simulink model "SildeModel_control"  (R2022b)
settings: Solver=ode4  StartTime=0.0  StopTime=t_total  FixedStep=sim_dt  RelTol=1e-3  EnableMultiTasking=on
InitFcn:
  | InitialCondition
values from neighbouring files (symbols this model uses):
  eps1 = 1e-4    (= 0.0001)    [InitialCondition.m]    (also in precise_plot.m = eps1_list(k))
  I_B = diag([200, 250, 300])    [InitialCondition.m]
  I_B_REAL = I_B*1.05    [InitialCondition.m]
  lambda_max_J = max(eig(I_B))    [InitialCondition.m]
  mrp0 = [0.2, 0.3, -0.3]    [InitialCondition.m]
  MRP_last = MRP_SEQ(end,:)    [InitialCondition.m]
  MRP_REAL0 = MRP_REAL0'    [InitialCondition.m]
  sim_dt = 0.01    [InitialCondition.m]
  Tau_SEQ = [Tau_SEQ;   Tau_EXT]    [InitialCondition.m]
  w0 = w0(:)    [Gauss_opt_mrp.m]    (also in InitialCondition.m = [0; 0; 0])
settings Model: Creator=Administrator  LastModifiedBy=33592
settings DataIOCC: ExternalInput=[t, y]  LimitDataPoints=on  MaxDataPoints=15000  ReturnWorkspaceOutputs=off
settings OptimizationCC: LifeSpan=inf
settings DebuggingCC: MultiTaskCondExecSysMsg=warning  MultiTaskRateTransMsg=warning  UnconnectedInputMsg=warning  UnconnectedOutputMsg=warning  UnconnectedLineMsg=warning  AllowSymbolicDim=off  SFUnexpectedBacktrackingDiag=warning  SFNoUnconditionalDefaultTransitionDiag=warning  SFExecutionAtInitializationDiag=none  SFMachineParentedDataDiag=warning  ArithmeticOperatorsInVariantConditions=warning
settings ModelReferenceCC: EnableRefExpFcnMdlSchedulingChecks=on  PropagateSignalLabelsOutOfModel=off
settings SFSimCC: SimUseLocalCustomCode=off  CustomCodeUndefinedFunction=UseInterfaceOnly
settings RTWCC: RTWUseLocalCustomCode=off
settings CodeAppCC: StateflowObjectComments=on
settings GRTTargetCC: TargetLangStandard=C89/C90 (ANSI)
settings ConfigComp: CovMetricSettings=dw  CovSaveCumulativeToWorkspaceVar=on  CovSaveSingleToWorkspaceVar=on  CovExternalEMLEnable=off

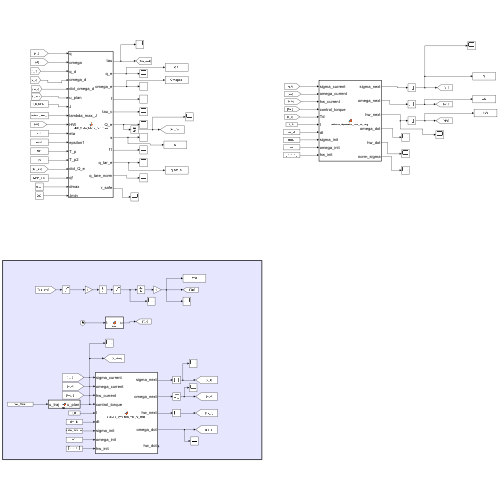
[thumbnail: Simulink's stored preview of the top-level diagram]
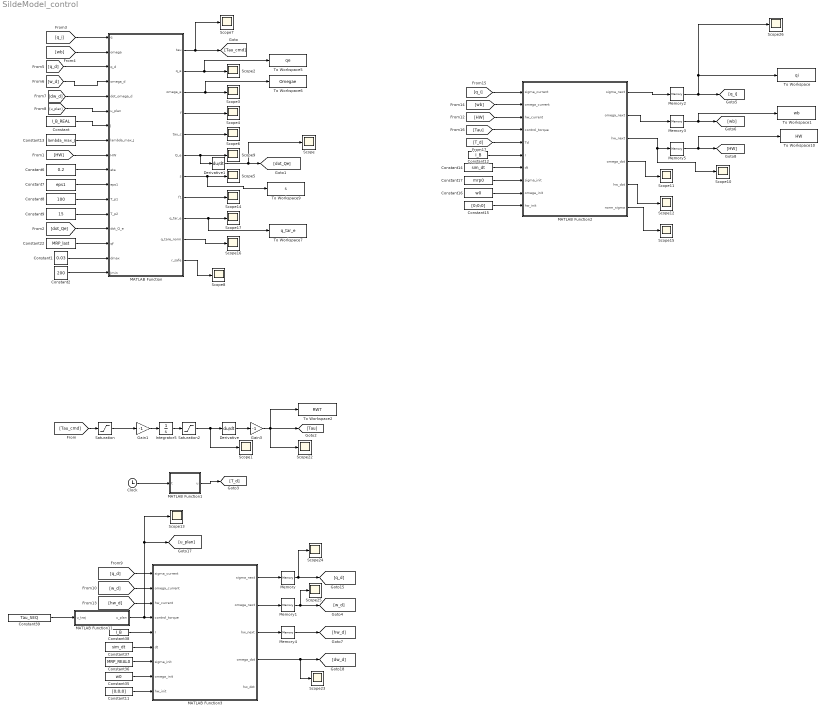
== system SildeModel_control ==
  Clock : Clock
  Constant : Constant  Value=I_B_REAL
  Constant1 : Constant  Value=0.03
  Constant11 : Constant  Value=[0;0;0]
  Constant12 : Constant  Value=I_B
  Constant13 : Constant  Value=lambda_max_J
  Constant14 : Constant  Value=sim_dt
  Constant15 : Constant  Value=[0;0;0]
  Constant16 : Constant  Value=w0
  Constant17 : Constant  Value=mrp0
  Constant2 : Constant  Value=200
  Constant22 : Constant  Value=MRP_last
  Constant35 : Constant  Value=w0
  Constant36 : Constant  Value=MRP_REAL0
  Constant37 : Constant  Value=sim_dt
  Constant38 : Constant  Value=I_B
  Constant39 : Constant  Value=Tau_SEQ
  Constant6 : Constant  Value=0.2
  Constant7 : Constant  Value=eps1
  Constant8 : Constant  Value=100
  Constant9 : Constant  Value=15
  Derivative : Derivative
  Derivative1 : Derivative
  Gain1 : Gain  Gain=-1
  Gain3 : Gain  Gain=-1
  Integrator5 : Integrator
  MATLAB Function : MATLAB Function  TreatAsAtomicUnit=on
  MATLAB Function1 : MATLAB Function  TreatAsAtomicUnit=on
  MATLAB Function11 : MATLAB Function  TreatAsAtomicUnit=on
  MATLAB Function2 : MATLAB Function  TreatAsAtomicUnit=on
  MATLAB Function3 : MATLAB Function  TreatAsAtomicUnit=on
  Memory{,1..5} (6 alike) : Memory
  Saturation : Saturate  UpperLimit=0.2  LowerLimit=-0.2
  Saturation2 : Saturate  UpperLimit=4  LowerLimit=-4
  Scope{,1..17,22..26} (23 alike) : Scope
  To Workspace : ToWorkspace  VariableName=qi  SampleTime=-1
  To Workspace1 : ToWorkspace  VariableName=wb  SampleTime=-1
  To Workspace10 : ToWorkspace  VariableName=HW  SampleTime=-1
  To Workspace2 : ToWorkspace  VariableName=RWT  SampleTime=-1
  To Workspace5 : ToWorkspace  VariableName=qe  SampleTime=-1
  To Workspace6 : ToWorkspace  VariableName=Omegae  SampleTime=-1
  To Workspace7 : ToWorkspace  VariableName=q_tar_e  SampleTime=-1
  To Workspace9 : ToWorkspace  VariableName=s  SampleTime=-1
  wires:
  MATLAB Function/1(tau) -> Scope7/1, [Tau_cmd]
  [q_i] -> MATLAB Function/1(q)
  [wb] -> MATLAB Function/2(omega)
  Constant/1 -> MATLAB Function/7(J)
  MATLAB Function/2(q_e) -> To Workspace5/1, Scope2/1
  Constant6/1 -> MATLAB Function/10(eta)
  Constant7/1 -> MATLAB Function/11(eps1)
  Constant8/1 -> MATLAB Function/12(T_p1)
  Constant9/1 -> MATLAB Function/13(T_p2)
  MATLAB Function/3(omega_e) -> To Workspace6/1, Scope3/1
  MATLAB Function/4(f) -> Scope4/1
  Constant13/1 -> MATLAB Function/8(lambda_max_J)
  MATLAB Function/7(s) -> To Workspace9/1, Scope5/1
  MATLAB Function/5(tau_c) -> Scope6/1
  MATLAB Function/6(Q_e) -> Derivative1/1, Scope9/1
  Clock/1 -> MATLAB Function1/1(t)
  MATLAB Function1/1(u) -> [T_d]
  MATLAB Function/8(f1) -> Scope14/1
  Constant22/1 -> MATLAB Function/15(qf)
  MATLAB Function/9(q_tar_e) -> To Workspace7/1, Scope17/1
  Gain1/1 -> Integrator5/1
  Constant35/1 -> MATLAB Function3/8(omega_init)
  Constant36/1 -> MATLAB Function3/7(sigma_init)
  Constant37/1 -> MATLAB Function3/6(dt)
  Constant38/1 -> MATLAB Function3/5(I)
  Constant39/1 -> MATLAB Function11/1(u_traj)
  MATLAB Function11/1(u_plan) -> Scope13/1, [u_plan], MATLAB Function3/4(control_torque)
  MATLAB Function3/1(sigma_next) -> Memory/1
  Memory/1 -> [q_d], Scope24/1
  MATLAB Function3/2(omega_next) -> Memory1/1
  Memory1/1 -> [w_d], Scope25/1
  MATLAB Function3/4(omega_dot) -> Scope23/1, [dw_d]
  MATLAB Function3/3(hw_next) -> Memory4/1
  Memory4/1 -> [hw_d]
  [q_d] -> MATLAB Function3/1(sigma_current)
  [w_d] -> MATLAB Function3/2(omega_current)
  [hw_d] -> MATLAB Function3/3(hw_current)
  Constant11/1 -> MATLAB Function3/9(hw_init)
  MATLAB Function2/1(sigma_next) -> Memory2/1
  Memory3/1 -> To Workspace1/1, [wb]
  Memory2/1 -> [q_i], To Workspace/1, Scope26/1
  MATLAB Function2/2(omega_next) -> Memory3/1
  MATLAB Function2/3(hw_next) -> Scope10/1, Memory5/1
  MATLAB Function2/4(omega_dot) -> Scope11/1
  MATLAB Function2/5(hw_dot) -> Scope12/1
  Memory5/1 -> To Workspace10/1, [HW]
  [HW] -> MATLAB Function2/3(hw_current)
  [wb] -> MATLAB Function2/2(omega_current)
  [q_i] -> MATLAB Function2/1(sigma_current)
  [Tau] -> MATLAB Function2/4(control_torque)
  [T_d] -> MATLAB Function2/5(Td)
  Constant12/1 -> MATLAB Function2/6(I)
  Constant14/1 -> MATLAB Function2/7(dt)
  Constant17/1 -> MATLAB Function2/8(sigma_init)
  Constant16/1 -> MATLAB Function2/9(omega_init)
  Constant15/1 -> MATLAB Function2/10(hw_init)
  [HW] -> MATLAB Function/9(HW)
  Derivative/1 -> Gain3/1
  Gain3/1 -> [Tau], To Workspace2/1, Scope22/1
  [u_plan] -> MATLAB Function/6(u_plan)
  [w_d] -> MATLAB Function/4(omega_d)
  [dw_d] -> MATLAB Function/5(dot_omega_d)
  [Tau_cmd] -> Saturation/1
  Saturation/1 -> Gain1/1
  Integrator5/1 -> Saturation2/1
  Derivative1/1 -> Scope/1, [dot_Qe]
  [dot_Qe] -> MATLAB Function/14(dot_Q_e)
  MATLAB Function/11(r_safe) -> Scope8/1
  Saturation2/1 -> Scope1/1, Derivative/1
  [q_d] -> MATLAB Function/3(q_d)
  Constant1/1 -> MATLAB Function/16(dmax)
  Constant2/1 -> MATLAB Function/17(Jmin)
  MATLAB Function2/6(norm_sigma) -> Scope15/1
  MATLAB Function/10(q_tare_norm) -> Scope16/1

== matlab function SildeModel_control/MATLAB Function3 ==
  data: sigma_current input; sigma_next output; omega_current input; hw_current input; control_torque input; I input; dt input; omega_next output; hw_next output; omega_dot output; sigma_init input; omega_init input; hw_init input; hw_dot output
function [sigma_next, omega_next, hw_next, omega_dot, hw_dot] = attitude_dynamics_mrp_rw_step(...
    sigma_current, omega_current, hw_current, control_torque, I, dt, sigma_init, omega_init, hw_init)
% 单步MRP姿态动力学计算（含反作用飞轮）- 用于Simulink
% 输入:
%   sigma_current - 当前MRP [σ1, σ2, σ3] (3×1)
%   omega_current - 当前角速度 [ω1, ω2, ω3] (3×1)
%   hw_current - 当前飞轮角动量 [hw1, hw2, hw3] (3×1)
%   control_torque - 控制力矩 [u1, u2, u3] (3×1) = -ḣw
%   I - 转动惯量矩阵 (3×3)
%   dt - 时间步长
%   reset - 重置信号，当为true时使用初始值
%   sigma_init - 初始MRP [σ1, σ2, σ3] (3×1)
%   omega_init - 初始角速度 [ω1, ω2, ω3] (3×1)
%   hw_init - 初始飞轮角动量 [hw1, hw2, hw3] (3×1)
% 输出:
%   sigma_next - 下一步MRP (3×1)
%   omega_next - 下一步角速度 (3×1)
%   hw_next - 下一步飞轮角动量 (3×1)
%   omega_dot - 当前角加速度 (3×1)
%   hw_dot - 当前飞轮角动量变化率 (3×1)
%   q_out - 对应的四元数 [q1, q2, q3, q4] (4×1)，用于参考
%   is_initialized - 初始化标志

    persistent initialized;
    
    % 第一次调用时初始化persistent变量
    if isempty(initialized)
        initialized = false;
    end
    
    % MRP动力学微分方程
    function dsigma = mrp_derivative(sigma, omega)
        % MRP运动学方程: σ̇ = G(σ)ω
        sigma_sq = sigma' * sigma;
        sigma_tilde = [0, -sigma(3), sigma(2); 
                      sigma(3), 0, -sigma(1);
                      -sigma(2), sigma(1), 0];
        
        G = 0.25 * ((1 - sigma_sq) * eye(3) + 2 * sigma_tilde + 2 * (sigma * sigma'));
        dsigma = G * omega;
    end

    % 角速度动力学微分方程（含飞轮）
    function dw = angular_velocity_derivative_rw(w, hw, u, I_matrix)
        % 欧拉动力学方程（含飞轮）: Iω̇ = u - ω × (Iω + hw)
        % 其中 u = -ḣw 是飞轮控制力矩
        dw = I_matrix \ (u - cross(w, I_matrix * w + hw));
    end

    % 飞轮角动量动力学微分方程
    function dhw = wheel_momentum_derivative(u)
        % 飞轮动力学: ḣw = -u
        % 其中 u = -ḣw 是飞轮控制力矩
        dhw = -u;
    end

    % 检查是否需要切换到影子MRP
    function sigma_checked = check_shadow_mrp(sigma)
        sigma_sq = sigma' * sigma;
        if sigma_sq > 1
            % 切换到影子MRP
            sigma_checked = -sigma / sigma_sq;
        else
            sigma_checked = sigma;
        end
    end

    % 处理初始化和重置
    if ~initialized
        % 使用初始值
        current_sigma = sigma_init(:);
        current_w = omega_init(:);
        current_hw = hw_init(:);
        initialized = true;
        is_initialized = true;
    else
        % 使用当前状态
        current_sigma = sigma_current(:);
        current_w = omega_current(:);
        current_hw = hw_current(:);
        is_initialized = false;
    end
    
    current_u = control_torque(:);
    
    % 计算角加速度和飞轮角动量变化率（用于输出）
    omega_dot = angular_velocity_derivative_rw(current_w, current_hw, current_u, I);
    hw_dot = wheel_momentum_derivative(current_u);
    
    % 使用四阶龙格-库塔法进行一步积分
    % k1
    k1_sigma = mrp_derivative(current_sigma, current_w);
    k1_w = angular_velocity_derivative_rw(current_w, current_hw, current_u, I);
    k1_hw = wheel_momentum_derivative(current_u);
    
    % k2
    k2_sigma = mrp_derivative(current_sigma + 0.5 * dt * k1_sigma, current_w + 0.5 * dt * k1_w);
    k2_w = angular_velocity_derivative_rw(current_w + 0.5 * dt * k1_w, current_hw + 0.5 * dt * k1_hw, current_u, I);
    k2_hw = wheel_momentum_derivative(current_u);
    
    % k3
    k3_sigma = mrp_derivative(current_sigma + 0.5 * dt * k2_sigma, current_w + 0.5 * dt * k2_w);
    k3_w = angular_velocity_derivative_rw(current_w + 0.5 * dt * k2_w, current_hw + 0.5 * dt * k2_hw, current_u, I);
    k3_hw = wheel_momentum_derivative(current_u);
    
    % k4
    k4_sigma = mrp_derivative(current_sigma + dt * k3_sigma, current_w + dt * k3_w);
    k4_w = angular_velocity_derivative_rw(current_w + dt * k3_w, current_hw + dt * k3_hw, current_u, I);
    k4_hw = wheel_momentum_derivative(current_u);
    
    % 更新MRP、角速度和飞轮角动量
    next_sigma = current_sigma + (dt / 6) * (k1_sigma + 2*k2_sigma + 2*k3_sigma + k4_sigma);
    next_w = current_w + (dt / 6) * (k1_w + 2*k2_w + 2*k3_w + k4_w);
    next_hw = current_hw + (dt / 6) * (k1_hw + 2*k2_hw + 2*k3_hw + k4_hw);
    
    % 检查并可能切换到影子MRP
    sigma_next = check_shadow_mrp(next_sigma);
    omega_next = next_w;
    hw_next = next_hw;

end

== matlab function SildeModel_control/MATLAB Function11 ==
  data: u_traj input; u_plan output
function u_plan  = fcn(u_traj)

persistent N

if isempty(N)
    N = 1;
end

u_traj = u_traj';
u_plan = u_traj(:,N);
N = N+1;

== matlab function SildeModel_control/MATLAB Function1 ==
  data: t input; u output
function u = fcn(t)

% if t > 0  && t<1
%     u = 0.06*[1 1 1]';
% else
%     u = 0.01*[sin(2*t), cos(1*t), cos(t+2)]';
% end

u = 0.01*[sin(2*t), cos(1*t), cos(t+2)]';

== matlab function SildeModel_control/MATLAB Function ==
  data: q input; omega input; q_d input; omega_d input; dot_omega_d input; u_plan input; tau output size=3; J input; lambda_max_J input; HW input; eta input; eps1 input; T_p1 input; T_p2 input; dot_Q_e input; q_e output size=3; omega_e output size=3; f output size=3; tau_c output size=3; Q_e output size=3; s output size=3; f1 output size=3; qf input size=3; q_tar_e output size=3; q_tare_norm output size=1; r_safe output size=1; dmax input; Jmin input
function [tau, q_e, omega_e, f, tau_c, Q_e, s, f1, q_tar_e, q_tare_norm, r_safe] = ...
    MRP_SlidingMode_Controller(q, omega, q_d, omega_d, dot_omega_d, u_plan,J, lambda_max_J, HW, ...
                                eta, eps1, T_p1, T_p2, dot_Q_e, qf, dmax, Jmin)
% MRP_SlidingMode_Controller
% 基于修正罗德里格斯参数(MRP)的预设时间滑模姿态控制器
%
% 输入:
%   q           - 当前姿态MRP (3×1)
%   q_d         - 期望姿态MRP (3×1)
%   omega       - 当前角速度 (3×1, 体坐标系)
%   omega_d     - 期望角速度 (3×1)
%   dot_omega_d - 期望角加速度 (3×1)
%   J           - 转动惯量矩阵 (3×3)
%   lambda_max_J- J的最大特征值 (标量)
%   hat_d       - 干扰估计 (3×1)
%   eta, epsilon, T_p, T_p2, a_d - 控制器参数
%
% 输出:
%   tau     - 控制力矩 (3×1)
%   q_e     - 姿态误差MRP (3×1)
%   omega_e - 角速度误差 (3×1)
%   f       - 前馈补偿项 (3×1)
%   tau_c   - 控制项 (3×1)
%   Q_e     - 滑模项函数值 (3×1)
%   s       - 滑模变量 (3×1)
%   dot_Q_e - Q_e的导数 (3×1)

%% ===== 常数计算 =====
c1 = pi / (eta * T_p1);

kappa1 = 1.2;    % alpha1 = kappa1 * alpha1_min
kappa2 = 1.2;    % alpha2 = kappa2 * alpha2_min
% ===== Derived constants =====


% 3. 计算均衡整定系数 Gamma
% 这里的指数项是 (1-eta)/(2-eta)
% 系数包含了 delta2, Tp1, Tp2 和 lambda_min
exponent = (1 - eta) / (2 - eta);

term_pre = (2 * dmax * T_p2) / (T_p1 * (Jmin^(1 - eta/2)));
Gamma = term_pre^(1 / (2 - eta));

% 4. 直接求解滑模面精度 eps2
eps2 = Gamma * (eps1^exponent);

% 5. 计算均衡后的最小理论增益 alpha_min
% 利用外环公式: alpha = (eta*Tp1*2^(-eta/2) / pi) * (eps2 / eps1^(1-eta))
alpha_star = (eta * T_p1 * 2^(-eta/2) / pi) * (eps2 / (eps1^(1 - eta)));


alpha1 = kappa1*alpha_star;
alpha2 = kappa2*alpha_star;

% k1 = 2^(1 + 1.5*eta);
% k2 = 2^(1 - eta/2);


% eps2 = (c1*k1hat/2^eta) * epsilon1^(1-eta);
% alpha1_min = (eta*T_p/pi) * 2^(-eta/2) * (eps2 / epsilon1^(1-eta));
% alpha1 = kappa1 * alpha1_min;
% alpha2_min = (delta2*eta*T_p2/pi) / ( (eps2/sqrt(2))^(1-eta) );
% alpha2 = kappa2 * alpha2_min;


k1 = 2^(1 + 1.5*eta)*(1 + alpha1);
k2 = 2^(1 - eta/2);

c2 = pi/ (eta*T_p2);
beta1 = 2^eta * (lambda_max_J/2)^(1 - eta/2)*(1+alpha2);
beta2 = (lambda_max_J/2)^(1 + eta/2);

epsilon2 = eps2;
% epsilon2 = eps2;


%% ===== 姿态误差与角速度误差 =====
q_e = mrp_error(q, q_d);
q_tar_e = mrp_error(q, qf);
C = mrp_to_dcm(q_e);                           % 误差DCM
omega_e = omega - C * omega_d;

%% ===== 计算 Q_e 和 s =====
r = norm(q_e);
Q_e = c1*k1*q_e / (r + eps1)^eta + c1*k2*q_e / (r + eps1)^(-eta);
s = omega_e + Q_e;

%% ===== 前馈补偿 f =====
f = -skew(omega)*(J*omega+HW) ...
    - J*C*dot_omega_d ...
    + J*skew(omega_e)*C*omega_d;
f1 = -skew(omega)*(J*omega+HW);

%% ===== dot_Q_e 推导实现 =====
r_safe = max(r, 1e-12);
% r_safe = r;
phi  = c1*( k1*(r + eps1)^(-eta) + k2*(r + eps1)^( eta) );
dphi = c1*eta*( -k1*(r + eps1)^(-eta-1) + k2*(r + eps1)^( eta-1) );

T_q = 0.5*((1 - q_e.'*q_e)*eye(3) + 2*skew(q_e) + 2*(q_e*q_e.'));
dot_q_e = T_q * omega_e;

scalar_proj = q_e.' * dot_q_e;
dot_Q_e = phi * dot_q_e + (dphi / r_safe) * scalar_proj * q_e;


% k_s = 0.1;

%% ===== 控制律 tau_c =====
norm_s = norm(s);
% tau_c = -c2*beta1 * s / (norm_s + epsilon1)^eta ...
%         -c2*beta2 * s / (norm_s + epsilon1)^(-eta) ...
%         - J * dot_Q_e;

tau_c = -c2*beta1 * s / (norm_s + epsilon2)^eta ...
        -c2*beta2 * s / (norm_s + epsilon2)^(-eta) ...
        - J * dot_Q_e;

% for i = 1:3
%     if norm(tau_c(i)) > 0.1
%         tau_c(i) = 0.1*sign(tau_c(i));
%     end
% end

%% ===== 最终控制力矩 =====
% tau = tau_c + u_plan;
tau = -f + tau_c;
% tau = +u_plan;

q_tare_norm = norm(q_tar_e);

end

%% ===== 辅助函数 =====
function q_e = mrp_error(q, q_d)
% MRP 姿态误差
denominator = 1 + (q_d'*q_d)*(q'*q) + 2*q_d'*q;
q_e = ( q_d*(q'*q - 1) + q*(1 - q_d'*q_d) - 2*skew(q_d)*q ) / denominator;
end

function C = mrp_to_dcm(q)
% 将MRP转换为方向余弦矩阵
q_norm_sq = q' * q;
denom = (1 + q_norm_sq)^2;
C = eye(3) + (8*skew(q)^2 - 4*(1 - q_norm_sq)*skew(q)) / denom;
end

function S = skew(v)
S = [0, -v(3), v(2);
     v(3), 0, -v(1);
     -v(2), v(1), 0];
end

== matlab function SildeModel_control/MATLAB Function2 ==
  settings: updateMethod=DISCRETE
  data: sigma_current input; sigma_next output; omega_current input; hw_current input; control_torque input; Td input; I input; dt input; omega_next output; hw_next output; omega_dot output; sigma_init input; omega_init input; hw_init input; hw_dot output; norm_sigma output
function [sigma_next, omega_next, hw_next, omega_dot, hw_dot,norm_sigma] = attitude_dynamics_mrp_rw_step(...
    sigma_current, omega_current, hw_current, control_torque, Td, I, dt, sigma_init, omega_init, hw_init)
% 单步MRP姿态动力学计算（含反作用飞轮）- 用于Simulink
% 输入:
%   sigma_current - 当前MRP [σ1, σ2, σ3] (3×1)
%   omega_current - 当前角速度 [ω1, ω2, ω3] (3×1)
%   hw_current - 当前飞轮角动量 [hw1, hw2, hw3] (3×1)
%   control_torque - 控制力矩 [u1, u2, u3] (3×1) = -ḣw
%   I - 转动惯量矩阵 (3×3)
%   dt - 时间步长
%   reset - 重置信号，当为true时使用初始值
%   sigma_init - 初始MRP [σ1, σ2, σ3] (3×1)
%   omega_init - 初始角速度 [ω1, ω2, ω3] (3×1)
%   hw_init - 初始飞轮角动量 [hw1, hw2, hw3] (3×1)
% 输出:
%   sigma_next - 下一步MRP (3×1)
%   omega_next - 下一步角速度 (3×1)
%   hw_next - 下一步飞轮角动量 (3×1)
%   omega_dot - 当前角加速度 (3×1)
%   hw_dot - 当前飞轮角动量变化率 (3×1)
%   q_out - 对应的四元数 [q1, q2, q3, q4] (4×1)，用于参考
%   is_initialized - 初始化标志

    persistent initialized;
    
    % 第一次调用时初始化persistent变量
    if isempty(initialized)
        initialized = false;
    end
    
    % MRP动力学微分方程
    function dsigma = mrp_derivative(sigma, omega)
        % MRP运动学方程: σ̇ = G(σ)ω
        sigma_sq = sigma' * sigma;
        sigma_tilde = [0, -sigma(3), sigma(2); 
                      sigma(3), 0, -sigma(1);
                      -sigma(2), sigma(1), 0];
        
        G = 0.25 * ((1 - sigma_sq) * eye(3) + 2 * sigma_tilde + 2 * (sigma * sigma'));
        dsigma = G * omega;
    end

    % 角速度动力学微分方程（含飞轮）
    function dw = angular_velocity_derivative_rw(w, hw, u, Td, I_matrix)
        % 欧拉动力学方程（含飞轮）: Iω̇ = u - ω × (Iω + hw)
        % 其中 u = -ḣw 是飞轮控制力矩
        dw = I_matrix \ (u+Td - cross(w, I_matrix * w + hw));
    end

    % 飞轮角动量动力学微分方程
    function dhw = wheel_momentum_derivative(u)
        % 飞轮动力学: ḣw = -u
        % 其中 u = -ḣw 是飞轮控制力矩
        dhw = -u;
    end

    % 检查是否需要切换到影子MRP
    function sigma_checked = check_shadow_mrp(sigma)
        sigma_sq = sigma' * sigma;
        if sigma_sq > 1
            % 切换到影子MRP
            sigma_checked = -sigma / sigma_sq;
        else
            sigma_checked = sigma;
        end
    end

    % 处理初始化和重置
    if ~initialized
        % 使用初始值
        current_sigma = sigma_init(:);
        current_w = omega_init(:);
        current_hw = hw_init(:);
        initialized = true;
        is_initialized = true;
    else
        % 使用当前状态
        current_sigma = sigma_current(:);
        current_w = omega_current(:);
        current_hw = hw_current(:);
        is_initialized = false;
    end
    
    current_u = control_torque(:);
    
    % 计算角加速度和飞轮角动量变化率（用于输出）
    omega_dot = angular_velocity_derivative_rw(current_w, current_hw, current_u, Td, I);
    hw_dot = wheel_momentum_derivative(current_u);
    
    % 使用四阶龙格-库塔法进行一步积分
    % k1
    k1_sigma = mrp_derivative(current_sigma, current_w);
    k1_w = angular_velocity_derivative_rw(current_w, current_hw, current_u, Td, I);
    k1_hw = wheel_momentum_derivative(current_u);
    
    % k2
    k2_sigma = mrp_derivative(current_sigma + 0.5 * dt * k1_sigma, current_w + 0.5 * dt * k1_w);
    k2_w = angular_velocity_derivative_rw(current_w + 0.5 * dt * k1_w, current_hw + 0.5 * dt * k1_hw, current_u, Td, I);
    k2_hw = wheel_momentum_derivative(current_u);
    
    % k3
    k3_sigma = mrp_derivative(current_sigma + 0.5 * dt * k2_sigma, current_w + 0.5 * dt * k2_w);
    k3_w = angular_velocity_derivative_rw(current_w + 0.5 * dt * k2_w, current_hw + 0.5 * dt * k2_hw, current_u, Td, I);
    k3_hw = wheel_momentum_derivative(current_u);
    
    % k4
    k4_sigma = mrp_derivative(current_sigma + dt * k3_sigma, current_w + dt * k3_w);
    k4_w = angular_velocity_derivative_rw(current_w + dt * k3_w, current_hw + dt * k3_hw, current_u, Td, I);
    k4_hw = wheel_momentum_derivative(current_u);
    
    % 更新MRP、角速度和飞轮角动量
    next_sigma = current_sigma + (dt / 6) * (k1_sigma + 2*k2_sigma + 2*k3_sigma + k4_sigma);
    next_w = current_w + (dt / 6) * (k1_w + 2*k2_w + 2*k3_w + k4_w);
    next_hw = current_hw + (dt / 6) * (k1_hw + 2*k2_hw + 2*k3_hw + k4_hw);
    
    % 检查并可能切换到影子MRP
    sigma_next = check_shadow_mrp(next_sigma);
    omega_next = next_w;
    hw_next = next_hw;
    norm_sigma = norm(sigma_next);

end
